simulink model "triplex_12B_with_contracts_PP"  (R2019b)
settings: Solver=FixedStepDiscrete  StartTime=0.0  StopTime=10.0  FixedStep=0.100000  RelTol=1e-3  EnableMultiTasking=on
model workspace (MAT data in the model file):
  ContractValidatorBlocksMap = containers.Map
  ContractValidatorBlocksMap.serialization.keys = {'triplex_12B/triplex_12B_TriplexSignalMonitorSpec/validator', 'triplex_12B_with_contracts/triplex_12B_TriplexSignalMonitorSpec/validator'}
  ContractValidatorBlocksMap.serialization.values{1}.block = 'triplex_12B/triplex_12B_TriplexSignalMonitorSpec/validator'
  ContractValidatorBlocksMap.serialization.values{1}.assumePorts = 1
  ContractValidatorBlocksMap.serialization.values{1}.guaranteePorts = 6
  ContractValidatorBlocksMap.serialization.values{1}.modeBlocksPorts = 0
  ContractValidatorBlocksMap.serialization.values{1}.portHandles.Inport = [1173.00195312 1174.00195312 1175.00195312 1176.00195312 1177.00195312 1178.00195312 1179.00195312]
  ContractValidatorBlocksMap.serialization.values{1}.portHandles.Outport = 1180.00195312
  ContractValidatorBlocksMap.serialization.values{1}.portHandles.Enable = []
  ContractValidatorBlocksMap.serialization.values{1}.portHandles.Trigger = []
  ContractValidatorBlocksMap.serialization.values{1}.portHandles.State = []
  ContractValidatorBlocksMap.serialization.values{1}.portHandles.LConn = []
  ContractValidatorBlocksMap.serialization.values{1}.portHandles.RConn = []
  ContractValidatorBlocksMap.serialization.values{1}.portHandles.Ifaction = []
  ContractValidatorBlocksMap.serialization.values{1}.portHandles.Reset = []
  ContractValidatorBlocksMap.serialization.values{1}.portConnectivity(1).Type = '1'
  ContractValidatorBlocksMap.serialization.values{1}.portConnectivity(1).Position = [365 -135]
  ContractValidatorBlocksMap.serialization.values{1}.portConnectivity(1).SrcBlock = 5288.00085449
  ContractValidatorBlocksMap.serialization.values{1}.portConnectivity(1).SrcPort = 0
  ContractValidatorBlocksMap.serialization.values{1}.portConnectivity(1).DstBlock = []
  ContractValidatorBlocksMap.serialization.values{1}.portConnectivity(1).DstPort = []
  ContractValidatorBlocksMap.serialization.values{1}.portConnectivity(2).Type = '2'
  ContractValidatorBlocksMap.serialization.values{1}.portConnectivity(2).Position = [365 -65]
  ContractValidatorBlocksMap.serialization.values{1}.portConnectivity(2).SrcBlock = 600.002807617
  ContractValidatorBlocksMap.serialization.values{1}.portConnectivity(2).SrcPort = 0
  ContractValidatorBlocksMap.serialization.values{1}.portConnectivity(2).DstBlock = []
  ContractValidatorBlocksMap.serialization.values{1}.portConnectivity(2).DstPort = []
  ContractValidatorBlocksMap.serialization.values{1}.portConnectivity(3).Type = '3'
  ContractValidatorBlocksMap.serialization.values{1}.portConnectivity(3).Position = [365 5]
  ContractValidatorBlocksMap.serialization.values{1}.portConnectivity(3).SrcBlock = 604.003051758
  ContractValidatorBlocksMap.serialization.values{1}.portConnectivity(3).SrcPort = 0
  ContractValidatorBlocksMap.serialization.values{1}.portConnectivity(3).DstBlock = []
  ContractValidatorBlocksMap.serialization.values{1}.portConnectivity(3).DstPort = []
  ContractValidatorBlocksMap.serialization.values{1}.portConnectivity(4).Type = '4'
  ContractValidatorBlocksMap.serialization.values{1}.portConnectivity(4).Position = [365 75]
  ContractValidatorBlocksMap.serialization.values{1}.portConnectivity(4).SrcBlock = 608.003051758
  ContractValidatorBlocksMap.serialization.values{1}.portConnectivity(4).SrcPort = 0
  ContractValidatorBlocksMap.serialization.values{1}.portConnectivity(4).DstBlock = []
  ContractValidatorBlocksMap.serialization.values{1}.portConnectivity(4).DstPort = []
  ContractValidatorBlocksMap.serialization.values{1}.portConnectivity(5).Type = '5'
  ContractValidatorBlocksMap.serialization.values{1}.portConnectivity(5).Position = [365 145]
  ContractValidatorBlocksMap.serialization.values{1}.portConnectivity(5).SrcBlock = 612.003051758
  ContractValidatorBlocksMap.serialization.values{1}.portConnectivity(5).SrcPort = 0
  ContractValidatorBlocksMap.serialization.values{1}.portConnectivity(5).DstBlock = []
  ContractValidatorBlocksMap.serialization.values{1}.portConnectivity(5).DstPort = []
  ContractValidatorBlocksMap.serialization.values{1}.portConnectivity(6).Type = '6'
  ContractValidatorBlocksMap.serialization.values{1}.portConnectivity(6).Position = [365 215]
  ContractValidatorBlocksMap.serialization.values{1}.portConnectivity(6).SrcBlock = 616.003051758
  ContractValidatorBlocksMap.serialization.values{1}.portConnectivity(6).SrcPort = 0
  ContractValidatorBlocksMap.serialization.values{1}.portConnectivity(6).DstBlock = []
  ContractValidatorBlocksMap.serialization.values{1}.portConnectivity(6).DstPort = []
  ContractValidatorBlocksMap.serialization.values{1}.portConnectivity(7).Type = '7'
  ContractValidatorBlocksMap.serialization.values{1}.portConnectivity(7).Position = [365 285]
  ContractValidatorBlocksMap.serialization.values{1}.portConnectivity(7).SrcBlock = 620.003051758
  ContractValidatorBlocksMap.serialization.values{1}.portConnectivity(7).SrcPort = 0
  ContractValidatorBlocksMap.serialization.values{1}.portConnectivity(7).DstBlock = []
  ContractValidatorBlocksMap.serialization.values{1}.portConnectivity(7).DstPort = []
  ContractValidatorBlocksMap.serialization.values{1}.portConnectivity(8).Type = '1'
  ContractValidatorBlocksMap.serialization.values{1}.portConnectivity(8).Position = [500 75]
  ContractValidatorBlocksMap.serialization.values{1}.portConnectivity(8).SrcBlock = []
  ContractValidatorBlocksMap.serialization.values{1}.portConnectivity(8).SrcPort = []
  ContractValidatorBlocksMap.serialization.values{1}.portConnectivity(8).DstBlock = 884.002807617
  ContractValidatorBlocksMap.serialization.values{1}.portConnectivity(8).DstPort = 0
  ContractValidatorBlocksMap.serialization.values{2}.block = 'triplex_12B_with_contracts/triplex_12B_TriplexSignalMonitorSpec/validator'
  ContractValidatorBlocksMap.serialization.values{2}.assumePorts = 0
  ContractValidatorBlocksMap.serialization.values{2}.guaranteePorts = 6
  ContractValidatorBlocksMap.serialization.values{2}.modeBlocksPorts = 0
  ContractValidatorBlocksMap.serialization.values{2}.portHandles.Inport = [2851.00195312 2852.0020752 2853.0020752 2854.00195312 2855.0020752 2856.00195312]
  ContractValidatorBlocksMap.serialization.values{2}.portHandles.Outport = 2857.0020752
  ContractValidatorBlocksMap.serialization.values{2}.portHandles.Enable = []
  ContractValidatorBlocksMap.serialization.values{2}.portHandles.Trigger = []
  ContractValidatorBlocksMap.serialization.values{2}.portHandles.State = []
  ContractValidatorBlocksMap.serialization.values{2}.portHandles.LConn = []
  ContractValidatorBlocksMap.serialization.values{2}.portHandles.RConn = []
  ContractValidatorBlocksMap.serialization.values{2}.portHandles.Ifaction = []
  ContractValidatorBlocksMap.serialization.values{2}.portHandles.Reset = []
  ContractValidatorBlocksMap.serialization.values{2}.portConnectivity(1).Type = '1'
  ContractValidatorBlocksMap.serialization.values{2}.portConnectivity(1).Position = [14780 -135]
  ContractValidatorBlocksMap.serialization.values{2}.portConnectivity(1).SrcBlock = 1443.00415039
  ContractValidatorBlocksMap.serialization.values{2}.portConnectivity(1).SrcPort = 0
  ContractValidatorBlocksMap.serialization.values{2}.portConnectivity(1).DstBlock = []
  ContractValidatorBlocksMap.serialization.values{2}.portConnectivity(1).DstPort = []
  ContractValidatorBlocksMap.serialization.values{2}.portConnectivity(2).Type = '2'
  ContractValidatorBlocksMap.serialization.values{2}.portConnectivity(2).Position = [14780 -50]
  ContractValidatorBlocksMap.serialization.values{2}.portConnectivity(2).SrcBlock = 1423.00378418
  ContractValidatorBlocksMap.serialization.values{2}.portConnectivity(2).SrcPort = 0
  ContractValidatorBlocksMap.serialization.values{2}.portConnectivity(2).DstBlock = []
  ContractValidatorBlocksMap.serialization.values{2}.portConnectivity(2).DstPort = []
  ContractValidatorBlocksMap.serialization.values{2}.portConnectivity(3).Type = '3'
  ContractValidatorBlocksMap.serialization.values{2}.portConnectivity(3).Position = [14780 35]
  ContractValidatorBlocksMap.serialization.values{2}.portConnectivity(3).SrcBlock = 1435.00390625
  ContractValidatorBlocksMap.serialization.values{2}.portConnectivity(3).SrcPort = 0
  ContractValidatorBlocksMap.serialization.values{2}.portConnectivity(3).DstBlock = []
  ContractValidatorBlocksMap.serialization.values{2}.portConnectivity(3).DstPort = []
  ContractValidatorBlocksMap.serialization.values{2}.portConnectivity(4).Type = '4'
  ContractValidatorBlocksMap.serialization.values{2}.portConnectivity(4).Position = [14780 120]
  ContractValidatorBlocksMap.serialization.values{2}.portConnectivity(4).SrcBlock = 1439.00305176
  ContractValidatorBlocksMap.serialization.values{2}.portConnectivity(4).SrcPort = 0
  ContractValidatorBlocksMap.serialization.values{2}.portConnectivity(4).DstBlock = []
  ContractValidatorBlocksMap.serialization.values{2}.portConnectivity(4).DstPort = []
  ContractValidatorBlocksMap.serialization.values{2}.portConnectivity(5).Type = '5'
  ContractValidatorBlocksMap.serialization.values{2}.portConnectivity(5).Position = [14780 205]
  ContractValidatorBlocksMap.serialization.values{2}.portConnectivity(5).SrcBlock = 1427.00415039
  ContractValidatorBlocksMap.serialization.values{2}.portConnectivity(5).SrcPort = 0
  ContractValidatorBlocksMap.serialization.values{2}.portConnectivity(5).DstBlock = []
  ContractValidatorBlocksMap.serialization.values{2}.portConnectivity(5).DstPort = []
  ContractValidatorBlocksMap.serialization.values{2}.portConnectivity(6).Type = '6'
  ContractValidatorBlocksMap.serialization.values{2}.portConnectivity(6).Position = [14780 290]
  ContractValidatorBlocksMap.serialization.values{2}.portConnectivity(6).SrcBlock = 1431.00537109
  ContractValidatorBlocksMap.serialization.values{2}.portConnectivity(6).SrcPort = 0
  ContractValidatorBlocksMap.serialization.values{2}.portConnectivity(6).DstBlock = []
  ContractValidatorBlocksMap.serialization.values{2}.portConnectivity(6).DstPort = []
  ContractValidatorBlocksMap.serialization.values{2}.portConnectivity(7).Type = '1'
  ContractValidatorBlocksMap.serialization.values{2}.portConnectivity(7).Position = [14915 80]
  ContractValidatorBlocksMap.serialization.values{2}.portConnectivity(7).SrcBlock = []
  ContractValidatorBlocksMap.serialization.values{2}.portConnectivity(7).SrcPort = []
  ContractValidatorBlocksMap.serialization.values{2}.portConnectivity(7).DstBlock = 2601.0020752
  ContractValidatorBlocksMap.serialization.values{2}.portConnectivity(7).DstPort = 0
  ContractValidatorBlocksMap.serialization.uniformity = 0
  ContractValidatorBlocksMap.serialization.keyType = 'char'
  ContractValidatorBlocksMap.serialization.valueType = 'any'
  already_pp = 1
  compositionalMap.analysisNames = {'triplex_12B_with_contracts_PP/TriplexMonitorNoFail'}
  compositionalMap.compositionalOptions = {{''}}
  compositionalMap.selectedOptions = 1
  maskControlsMap = containers.Map
  maskControlsMap.serialization.keys = {'triplex_12B_with_contracts_PP/triplex_12B_TriplexSignalMonitorSpec/TSM_minus_004'}
  maskControlsMap.serialization.values = {{'Display_counter_example_as_signals', 'Display_counter_example_as_tables', 'Display_counter_example_as_HTML_tables', 'Generate_an_outer_model_for_the_counter_example', 'Generate_an_inner_model_for_the_counter_example'}}
  maskControlsMap.serialization.uniformity = 0
  maskControlsMap.serialization.keyType = 'char'
  maskControlsMap.serialization.valueType = 'any'
  nodeNameToBlockNameMap : containers.Map (value not decoded)
  verificationResults : object (value not decoded)
undefined symbols (not defined in the file): contractAfterSimulation, contractBeforeSimulation, ContractBlock, ContractGuaranteeBlock, ContractValidatorBlock, saveValidatorParameters
(part 1 of 2)
settings Model: Creator=elliocm  LastModifiedBy=hbourbou
settings DataIOCC: LimitDataPoints=on  SaveFormat=StructureWithTime  SignalLoggingSaveFormat=ModelDataLogs  ReturnWorkspaceOutputs=off
settings OptimizationCC: ExpressionDepthLimit=2147483647  LifeSpan=inf
settings DebuggingCC: AlgebraicLoopMsg=error  ArtificialAlgebraicLoopMsg=error  UnderspecifiedInitializationDetection=Classic  MergeDetectMultiDrivingBlocksExec=none  SolverPrmCheckMsg=warning  MultiTaskDSMMsg=warning  MultiTaskCondExecSysMsg=none  SingleTaskRateTransMsg=error  StateNameClashWarn=warning  SFUnexpectedBacktrackingDiag=warning  SFNoUnconditionalDefaultTransitionDiag=warning  SFExecutionAtInitializationDiag=none  ArithmeticOperatorsInVariantConditions=warning
settings HardwareCC: ProdBitPerPointer=32  ProdBitPerSizeT=32  ProdBitPerPtrDiffT=32  ProdLargestAtomicFloat=None  ProdIntDivRoundTo=Undefined  ProdEndianess=Unspecified  ProdWordSize=32  ProdHWDeviceType=32-bit Generic
settings ModelReferenceCC: PropagateSignalLabelsOutOfModel=off
settings SFSimCC: SimUseLocalCustomCode=off  CustomCodeUndefinedFunction=UseInterfaceOnly
settings RTWCC: RTWUseLocalCustomCode=off
settings CodeAppCC: StateflowObjectComments=on
settings GRTTargetCC: TargetLangStandard=C89/C90 (ANSI)  GeneratePreprocessorConditionals=Disable all
settings ConfigComp: CovMetricSettings=dw  CovHtmlReporting=on  CovSaveCumulativeToWorkspaceVar=on  CovSaveSingleToWorkspaceVar=on  CovExternalEMLEnable=off

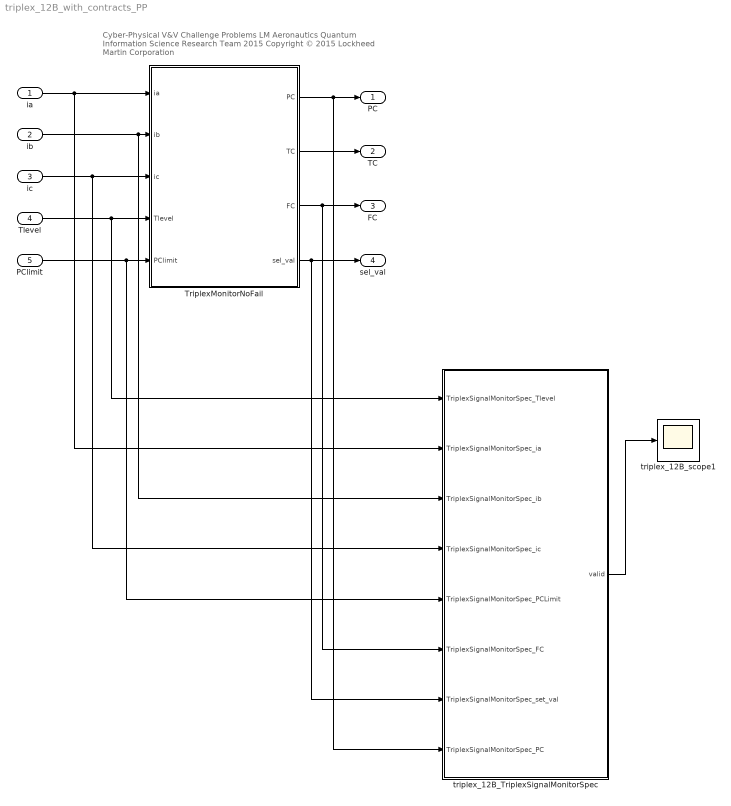
== system triplex_12B_with_contracts_PP ==
  note: Cyber-Physical V&V Challenge Problems
      | LM Aeronautics Quantum Information Science Research Team 2015
      | Copyright © 2015 Lockheed Martin Corporation
  ia : Inport  OutDataTypeStr=double
  ib : Inport  Port=2  OutDataTypeStr=double
  ic : Inport  Port=3  OutDataTypeStr=double
  Tlevel : Inport  Port=4  OutDataTypeStr=double
  PClimit : Inport  Port=5  OutDataTypeStr=int32
  TriplexMonitorNoFail : Subsystem  TreatAsAtomicUnit=on
  triplex_12B_TriplexSignalMonitorSpec : Subsystem  TreatAsAtomicUnit=on  mask(ContractBlock){ContractBlockType=ContractBlock}
      mask init:
      | set_param(gcb, 'LinkStatus', 'none');
      mask DialogControl DescTextVar Prompt: Contract block
      mask Display:
      | text(0.5, 0.5, '{\bf\fontsize{20}Contract}', 'hor', 'center', 'texmode','on');
      | blocks = find_system(gcb, 'LookUnderMasks','all', 'SearchDepth',1,'BlockType','Inport');
      | for i = 1 : length(blocks)
      |     blockName = get_param(blocks(i), 'Name');
      |     [path, blockName] = fileparts(char(blockName));
      |     port_label('input', i, blockName);
      | end
      | 
      | blocks = find_system(gcb, 'LookUnderMasks','all', 'SearchDepth',1,'BlockType','Outport');
      | for i = 1 : length(blocks)
      |     blockName = get_param(blocks(i), 'Name');
      |     [path, blockName] = fileparts(char(blockName));
      |     port_label('output', i, blockName);
      | end
  triplex_12B_scope1 : Scope
  PC : Outport  VectorParamsAs1DForOutWhenUnconnected=off
  TC : Outport  Port=2  VectorParamsAs1DForOutWhenUnconnected=off
  FC : Outport  Port=3  VectorParamsAs1DForOutWhenUnconnected=off
  sel_val : Outport  Port=4  VectorParamsAs1DForOutWhenUnconnected=off
  wires:
  ia/1 -> TriplexMonitorNoFail/1(ia), triplex_12B_TriplexSignalMonitorSpec/2(TriplexSignalMonitorSpec_ia)
  ib/1 -> TriplexMonitorNoFail/2(ib), triplex_12B_TriplexSignalMonitorSpec/3(TriplexSignalMonitorSpec_ib)
  Tlevel/1 -> TriplexMonitorNoFail/4(Tlevel), triplex_12B_TriplexSignalMonitorSpec/1(TriplexSignalMonitorSpec_Tlevel)
  PClimit/1 -> TriplexMonitorNoFail/5(PClimit), triplex_12B_TriplexSignalMonitorSpec/5(TriplexSignalMonitorSpec_PCLimit)
  TriplexMonitorNoFail/2(TC) -> TC/1
  TriplexMonitorNoFail/1(PC) -> PC/1, triplex_12B_TriplexSignalMonitorSpec/8(TriplexSignalMonitorSpec_PC)
  TriplexMonitorNoFail/4(sel_val) -> sel_val/1, triplex_12B_TriplexSignalMonitorSpec/7(TriplexSignalMonitorSpec_set_val)
  ic/1 -> TriplexMonitorNoFail/3(ic), triplex_12B_TriplexSignalMonitorSpec/4(TriplexSignalMonitorSpec_ic)
  TriplexMonitorNoFail/3(FC) -> FC/1, triplex_12B_TriplexSignalMonitorSpec/6(TriplexSignalMonitorSpec_FC)
  triplex_12B_TriplexSignalMonitorSpec/1(valid) -> triplex_12B_scope1/1

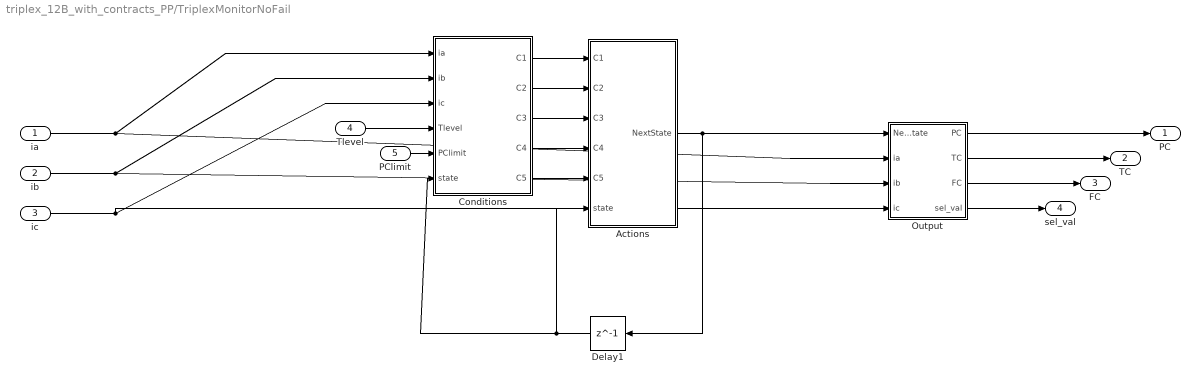
== system triplex_12B_with_contracts_PP/TriplexMonitorNoFail ==
  ia : Inport
  ib : Inport  Port=2
  ic : Inport  Port=3
  Tlevel : Inport  Port=4
  PClimit : Inport  Port=5
  Actions : Subsystem  TreatAsAtomicUnit=on
  Conditions : Subsystem  TreatAsAtomicUnit=on
  Delay1 : Delay  DelayLength=1  InitialCondition=0
  Output : Subsystem  TreatAsAtomicUnit=on
  PC : Outport  VectorParamsAs1DForOutWhenUnconnected=off
  TC : Outport  Port=2  VectorParamsAs1DForOutWhenUnconnected=off
  FC : Outport  Port=3  VectorParamsAs1DForOutWhenUnconnected=off
  sel_val : Outport  Port=4  VectorParamsAs1DForOutWhenUnconnected=off
  wires:
  Conditions/2(C2) -> Actions/2(C2)
  Conditions/5(C5) -> Actions/5(C5)
  Conditions/1(C1) -> Actions/1(C1)
  Conditions/4(C4) -> Actions/4(C4)
  Conditions/3(C3) -> Actions/3(C3)
  Tlevel/1 -> Conditions/4(Tlevel)
  PClimit/1 -> Conditions/5(PClimit)
  Output/2(TC) -> TC/1
  Output/1(PC) -> PC/1
  Output/3(FC) -> FC/1
  Actions/1(NextState) -> Delay1/1, Output/1(NextState)
  Delay1/1 -> Actions/6(state), Conditions/6(state)
  ia/1 -> Conditions/1(ia), Output/2(ia)
  ib/1 -> Conditions/2(ib), Output/3(ib)
  ic/1 -> Conditions/3(ic), Output/4(ic)
  Output/4(sel_val) -> sel_val/1

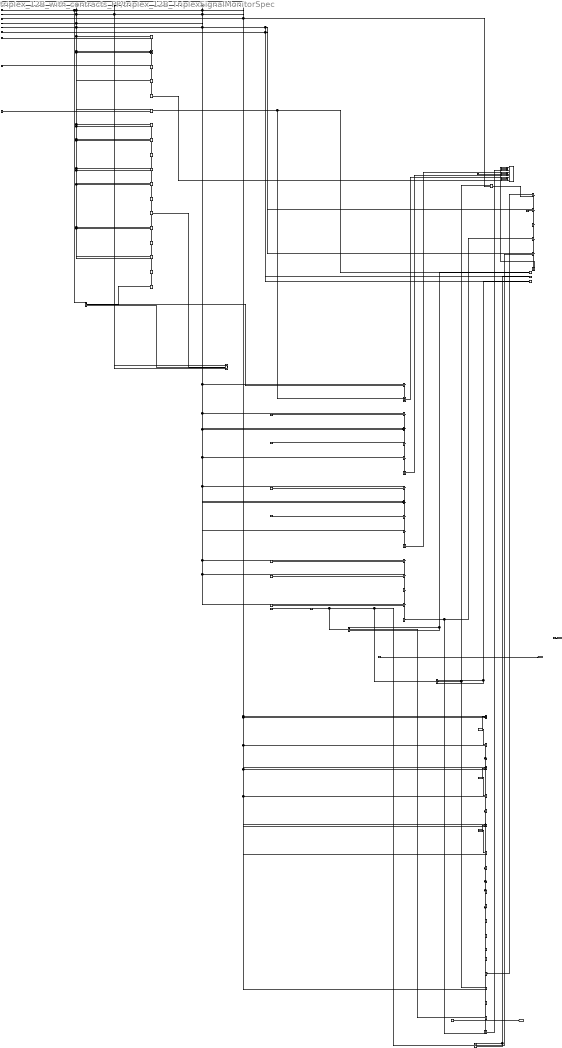
== system triplex_12B_with_contracts_PP/triplex_12B_TriplexSignalMonitorSpec ==
  TriplexSignalMonitorSpec_Tlevel : Inport  OutDataTypeStr=double
  TriplexSignalMonitorSpec_ia : Inport  Port=2  OutDataTypeStr=double
  TriplexSignalMonitorSpec_ib : Inport  Port=3  OutDataTypeStr=double
  TriplexSignalMonitorSpec_ic : Inport  Port=4  OutDataTypeStr=double
  TriplexSignalMonitorSpec_PCLimit : Inport  Port=5
  TriplexSignalMonitorSpec_FC : Inport  Port=6
  TriplexSignalMonitorSpec_set_val : Inport  Port=7  OutDataTypeStr=double
  TriplexSignalMonitorSpec_PC : Inport  Port=8
  Arrow_xxTriplexS_443436564_ec_35_ni_0 : Delay  DelayLength=1  InitialCondition=1
  C1_operator : RelationalOperator  Operator=>  OutDataTypeStr=boolean  RndMeth=Simplest
  C2_operator : RelationalOperator  Operator=>  OutDataTypeStr=boolean  RndMeth=Simplest
  C3_operator : RelationalOperator  Operator=>  OutDataTypeStr=boolean  RndMeth=Simplest
  PRE_xxTriplexSignalMonitorSpec_37 : Delay  DelayLength=1  InitialCondition=0
  PRE_xxTriplexSignalMonitorSpec_40 : Delay  DelayLength=1  InitialCondition=0
  PRE_xxTriplexSignalMonitorSpec_46 : Delay  DelayLength=1  InitialCondition=0
  TSM_minus_001 : Subsystem  TreatAsAtomicUnit=on  mask(ContractGuaranteeBlock){ContractBlockType=ContractGuaranteeBlock}
      mask init:
      | set_param(gcb, 'LinkStatus', 'none');
      mask DialogControl DescTextVar Prompt: Guarantee block
  TSM_minus_002 : Subsystem  TreatAsAtomicUnit=on  mask(ContractGuaranteeBlock){ContractBlockType=ContractGuaranteeBlock}
      mask init:
      | set_param(gcb, 'LinkStatus', 'none');
      mask DialogControl DescTextVar Prompt: Guarantee block
  TSM_minus_003a : Subsystem  TreatAsAtomicUnit=on  mask(ContractGuaranteeBlock){ContractBlockType=ContractGuaranteeBlock}
      mask init:
      | set_param(gcb, 'LinkStatus', 'none');
      mask DialogControl DescTextVar Prompt: Guarantee block
  TSM_minus_003b : Subsystem  TreatAsAtomicUnit=on  mask(ContractGuaranteeBlock){ContractBlockType=ContractGuaranteeBlock}
      mask init:
      | set_param(gcb, 'LinkStatus', 'none');
      mask DialogControl DescTextVar Prompt: Guarantee block
  TSM_minus_003c : Subsystem  TreatAsAtomicUnit=on  mask(ContractGuaranteeBlock){ContractBlockType=ContractGuaranteeBlock}
      mask init:
      | set_param(gcb, 'LinkStatus', 'none');
      mask DialogControl DescTextVar Prompt: Guarantee block
  TSM_minus_004 : Subsystem  TreatAsAtomicUnit=on  mask(ContractGuaranteeBlock){ContractBlockType=ContractGuaranteeBlock}
      mask init:
      | set_param(gcb, 'LinkStatus', 'none');
      mask DialogControl DescTextVar Prompt: Guarantee block
      mask DialogControl Display_counter_example_as_signals Prompt: Display counter example as signals
      mask DialogControl Display_counter_example_as_signals Callback: displayCexSignals(1, 1);
      mask DialogControl Display_counter_example_as_tables Prompt: Display counter example as tables
      mask DialogControl Display_counter_example_as_tables Callback: displayCexTables(1, 1);
      mask DialogControl Display_counter_example_as_HTML_tables Prompt: Display counter example as HTML tables
      mask DialogControl Display_counter_example_as_HTML_tables Callback: displayCexHtmlTables(1, 1);
      mask DialogControl Generate_an_outer_model_for_the_counter_example Prompt: Generate an outer model for the counter example
      mask DialogControl Generate_an_outer_model_for_the_counter_example Callback: generateModelWithSignalBuilders(1, 1, 2);
      mask DialogControl Generate_an_inner_model_for_the_counter_example Prompt: Generate an inner model for the counter example
      mask DialogControl Generate_an_inner_model_for_the_counter_example Callback: generateModelWithSignalBuilders(1, 1, 1);
  abs_call : Subsystem  TreatAsAtomicUnit=on
  abs_call1 : Subsystem  TreatAsAtomicUnit=on
  abs_call11 : Subsystem  TreatAsAtomicUnit=on
  branch_10_IF : Switch  Criteria=u2 ~= 0
  branch_11_IF : Switch  Criteria=u2 ~= 0
  branch_12_IF : Switch  Criteria=u2 ~= 0
  branch_13_IF : Switch  Criteria=u2 ~= 0
  branch_9_IF : Switch  Criteria=u2 ~= 0
  failure_in_progress_operator : Logic  AllPortsSameDT=off  OutDataTypeStr=boolean
  failure_must_be_latched_operator : Logic  AllPortsSameDT=off  OutDataTypeStr=boolean
  miscompare_operator : Logic  Operator=OR  AllPortsSameDT=off  OutDataTypeStr=boolean
  no_fail_operator : RelationalOperator  Operator===  OutDataTypeStr=boolean  RndMeth=Simplest
  no_fail_rhs_2 : Constant  Value=0  OutDataTypeStr=int32
  single_fail_reported_operator : Logic  Operator=OR  AllPortsSameDT=off  OutDataTypeStr=boolean
  spec284_operator : Subsystem  TreatAsAtomicUnit=on
  spec292_operator : Subsystem  TreatAsAtomicUnit=on
  spec309_operator : Subsystem  TreatAsAtomicUnit=on
  spec326_operator : Subsystem  TreatAsAtomicUnit=on
  spec334_operator : Subsystem  TreatAsAtomicUnit=on
  spec351_operator : Subsystem  TreatAsAtomicUnit=on
  validator : M-S-Function  LoadFcn=saveValidatorParameters(gcb);  InitFcn=contractBeforeSimulation();  StopFcn=contractAfterSimulation();  FunctionName=contract  mask(ContractValidatorBlock){assumePorts=0, guaranteePorts=6, modePorts=0, ContractBlockType=ContractValidatorBlock, createInportsCheckbox=off}
      mask prompts: assumePorts "Assume ports     :"; guaranteePorts "Guarantee ports :"; modePorts "Mode ports        :"; createInportsCheckbox "Create inports and connect them automatically"
      mask init:
      | set_param(gcb,'LinkStatus','none');
      | contract_callback('inputs_callback',gcb);
      mask DialogControl DescTextVar Prompt: The validator block implements the following logic: <br> <br> <b>Sofar</b>(assume<sub>1</sub> <b>&#8743;</b> assume<sub>2</sub> <b>&#8743;</b> ... assume<sub>k</sub>) <b>&rarr;</b> (guarantee<sub>1</sub> <b>&#8743;</b> guarantee<sub>2</sub> <b>&#8743;</b> ... guarantee<sub>m</sub> <b>&#8743;</b>  mode<sub>1</sub> <b>&#8743;</b> mode<sub>2</sub> <b>&#8743;</b> ... <b>&#8743;</b> mode<sub>n</sub> )<br> where mode<sub>i</sub> = require<sub>i</sub> <b>&rarr;</b> ensure<sub>i</sub>
      mask Display:
      | color('black');
      | port_label('input',1,'guarantee');
      | port_label('input',2,'guarantee');
      | port_label('input',3,'guarantee');
      | port_label('input',4,'guarantee');
      | port_label('input',5,'guarantee');
      | port_label('input',6,'guarantee');
      | port_label('output',1,'valid');
  xxTriplexS_443436564_ec_35_ni_0_init : Constant  Value=0  OutDataTypeStr=boolean
  xxTriplexSignalMonitorSpec_10_operator : Sum  OutDataTypeStr=double
  xxTriplexSignalMonitorSpec_11_operator : Product  OutDataTypeStr=double
  xxTriplexSignalMonitorSpec_11_rhs_1 : Constant  Value=0.5  OutDataTypeStr=double
  xxTriplexSignalMonitorSpec_12_operator : RelationalOperator  Operator===  OutDataTypeStr=boolean  RndMeth=Simplest
  xxTriplexSignalMonitorSpec_13_operator : RelationalOperator  Operator===  OutDataTypeStr=boolean  RndMeth=Simplest
  xxTriplexSignalMonitorSpec_13_rhs_2 : Constant  Value=2  OutDataTypeStr=int32
  xxTriplexSignalMonitorSpec_14_operator : Logic  AllPortsSameDT=off  OutDataTypeStr=boolean
  xxTriplexSignalMonitorSpec_15_operator : RelationalOperator  Operator===  OutDataTypeStr=boolean  RndMeth=Simplest
  xxTriplexSignalMonitorSpec_16_operator : Logic  AllPortsSameDT=off  OutDataTypeStr=boolean
  xxTriplexSignalMonitorSpec_17_operator : Sum  Inputs=+-  OutDataTypeStr=double
  xxTriplexSignalMonitorSpec_19_operator : Sum  Inputs=+-  OutDataTypeStr=double
  xxTriplexSignalMonitorSpec_1_operator : Sum  OutDataTypeStr=double
  xxTriplexSignalMonitorSpec_21_operator : Sum  Inputs=+-  OutDataTypeStr=double
  xxTriplexSignalMonitorSpec_23_operator : RelationalOperator  Operator=<=  OutDataTypeStr=boolean  RndMeth=Simplest
  xxTriplexSignalMonitorSpec_24_operator : RelationalOperator  Operator=<=  OutDataTypeStr=boolean  RndMeth=Simplest
  xxTriplexSignalMonitorSpec_25_operator : Logic  AllPortsSameDT=off  OutDataTypeStr=boolean
  xxTriplexSignalMonitorSpec_26_operator : RelationalOperator  Operator=<=  OutDataTypeStr=boolean  RndMeth=Simplest
  xxTriplexSignalMonitorSpec_27_operator : RelationalOperator  Operator=<=  OutDataTypeStr=boolean  RndMeth=Simplest
  xxTriplexSignalMonitorSpec_28_operator : Logic  AllPortsSameDT=off  OutDataTypeStr=boolean
  xxTriplexSignalMonitorSpec_29_operator : Logic  Operator=OR  AllPortsSameDT=off  OutDataTypeStr=boolean
  xxTriplexSignalMonitorSpec_2_operator : Product  OutDataTypeStr=double
  xxTriplexSignalMonitorSpec_2_rhs_1 : Constant  Value=0.5  OutDataTypeStr=double
  xxTriplexSignalMonitorSpec_30_operator : RelationalOperator  Operator=<=  OutDataTypeStr=boolean  RndMeth=Simplest
  xxTriplexSignalMonitorSpec_31_operator : Logic  AllPortsSameDT=off  OutDataTypeStr=boolean
  xxTriplexSignalMonitorSpec_32_operator : RelationalOperator  Operator=<=  OutDataTypeStr=boolean  RndMeth=Simplest
  xxTriplexSignalMonitorSpec_33_operator : Logic  AllPortsSameDT=off  OutDataTypeStr=boolean
  xxTriplexSignalMonitorSpec_34_operator : Logic  Operator=OR  AllPortsSameDT=off  OutDataTypeStr=boolean
  xxTriplexSignalMonitorSpec_36_rhs : Constant  Value=0  OutDataTypeStr=Inherit: Inherit via back propagation
  xxTriplexSignalMonitorSpec_39_rhs : Constant  Value=0.0  OutDataTypeStr=double
  xxTriplexSignalMonitorSpec_3_operator : RelationalOperator  Operator===  OutDataTypeStr=boolean  RndMeth=Simplest
  xxTriplexSignalMonitorSpec_42_operator : RelationalOperator  Operator=>  OutDataTypeStr=boolean  RndMeth=Simplest
  xxTriplexSignalMonitorSpec_42_rhs_2 : Constant  Value=0  OutDataTypeStr=int32
  xxTriplexSignalMonitorSpec_43_operator : RelationalOperator  Operator=<=  OutDataTypeStr=boolean  RndMeth=Simplest
  xxTriplexSignalMonitorSpec_44_operator : Logic  AllPortsSameDT=off  OutDataTypeStr=boolean
  xxTriplexSignalMonitorSpec_45_operator : RelationalOperator  Operator=>  OutDataTypeStr=boolean  RndMeth=Simplest
  xxTriplexSignalMonitorSpec_47_rhs1 : Constant  Value=true  OutDataTypeStr=boolean
  xxTriplexSignalMonitorSpec_48_operator : RelationalOperator  Operator===  OutDataTypeStr=boolean  RndMeth=Simplest
  xxTriplexSignalMonitorSpec_48_rhs_2 : Constant  Value=4  OutDataTypeStr=int32
  xxTriplexSignalMonitorSpec_49_operator : RelationalOperator  Operator===  OutDataTypeStr=boolean  RndMeth=Simplest
  xxTriplexSignalMonitorSpec_49_rhs_2 : Constant  Value=2  OutDataTypeStr=int32
  xxTriplexSignalMonitorSpec_4_operator : RelationalOperator  Operator===  OutDataTypeStr=boolean  RndMeth=Simplest
  xxTriplexSignalMonitorSpec_4_rhs_2 : Constant  OutDataTypeStr=int32
  xxTriplexSignalMonitorSpec_50_operator : RelationalOperator  Operator===  OutDataTypeStr=boolean  RndMeth=Simplest
  xxTriplexSignalMonitorSpec_50_rhs_2 : Constant  OutDataTypeStr=int32
  xxTriplexSignalMonitorSpec_51_operator : Logic  Operator=OR  AllPortsSameDT=off  OutDataTypeStr=boolean
  xxTriplexSignalMonitorSpec_52_operator : Logic  Operator=NOT  AllPortsSameDT=off  OutDataTypeStr=boolean
  xxTriplexSignalMonitorSpec_53_operator : Logic  AllPortsSameDT=off  OutDataTypeStr=boolean
  xxTriplexSignalMonitorSpec_54_operator : Logic  AllPortsSameDT=off  OutDataTypeStr=boolean
  xxTriplexSignalMonitorSpec_55_operator : Logic  Operator=NOT  AllPortsSameDT=off  OutDataTypeStr=boolean
  xxTriplexSignalMonitorSpec_56_operator : Logic  AllPortsSameDT=off  OutDataTypeStr=boolean
  xxTriplexSignalMonitorSpec_57_operator : Logic  AllPortsSameDT=off  OutDataTypeStr=boolean
  xxTriplexSignalMonitorSpec_58_operator : Logic  Operator=NOT  AllPortsSameDT=off  OutDataTypeStr=boolean
  xxTriplexSignalMonitorSpec_59_operator : Logic  AllPortsSameDT=off  OutDataTypeStr=boolean
  xxTriplexSignalMonitorSpec_5_operator : RelationalOperator  Operator===  OutDataTypeStr=boolean  RndMeth=Simplest
  xxTriplexSignalMonitorSpec_60_operator : Logic  AllPortsSameDT=off  OutDataTypeStr=boolean
  xxTriplexSignalMonitorSpec_61_operator : Logic  Operator=OR  AllPortsSameDT=off  OutDataTypeStr=boolean
  xxTriplexSignalMonitorSpec_6_operator : Sum  OutDataTypeStr=double
  xxTriplexSignalMonitorSpec_7_operator : Product  OutDataTypeStr=double
  xxTriplexSignalMonitorSpec_7_rhs_1 : Constant  Value=0.5  OutDataTypeStr=double
  xxTriplexSignalMonitorSpec_8_operator : RelationalOperator  Operator===  OutDataTypeStr=boolean  RndMeth=Simplest
  xxTriplexSignalMonitorSpec_9_operator : RelationalOperator  Operator===  OutDataTypeStr=boolean  RndMeth=Simplest
  xxTriplexSignalMonitorSpec_9_rhs_2 : Constant  Value=4  OutDataTypeStr=int32
  valid : Outport
  wires:
  validator/1 -> valid/1
  xxTriplexSignalMonitorSpec_9_rhs_2/1 -> xxTriplexSignalMonitorSpec_9_operator/2
  xxTriplexSignalMonitorSpec_7_operator/1 -> xxTriplexSignalMonitorSpec_8_operator/2
  xxTriplexSignalMonitorSpec_6_operator/1 -> xxTriplexSignalMonitorSpec_7_operator/2
  xxTriplexSignalMonitorSpec_7_rhs_1/1 -> xxTriplexSignalMonitorSpec_7_operator/1
  xxTriplexSignalMonitorSpec_57_operator/1 -> xxTriplexSignalMonitorSpec_61_operator/2
  xxTriplexSignalMonitorSpec_60_operator/1 -> xxTriplexSignalMonitorSpec_61_operator/1
  xxTriplexSignalMonitorSpec_59_operator/1 -> xxTriplexSignalMonitorSpec_60_operator/1
  branch_9_IF/1 -> xxTriplexSignalMonitorSpec_5_operator/2
  xxTriplexSignalMonitorSpec_58_operator/1 -> xxTriplexSignalMonitorSpec_59_operator/1
  xxTriplexSignalMonitorSpec_56_operator/1 -> xxTriplexSignalMonitorSpec_57_operator/1
  xxTriplexSignalMonitorSpec_55_operator/1 -> xxTriplexSignalMonitorSpec_56_operator/2
  xxTriplexSignalMonitorSpec_52_operator/1 -> xxTriplexSignalMonitorSpec_54_operator/2
  xxTriplexSignalMonitorSpec_53_operator/1 -> xxTriplexSignalMonitorSpec_54_operator/1
  xxTriplexSignalMonitorSpec_49_operator/1 -> xxTriplexSignalMonitorSpec_51_operator/2
  xxTriplexSignalMonitorSpec_50_operator/1 -> xxTriplexSignalMonitorSpec_51_operator/1
  xxTriplexSignalMonitorSpec_50_rhs_2/1 -> xxTriplexSignalMonitorSpec_50_operator/2
  xxTriplexSignalMonitorSpec_4_rhs_2/1 -> xxTriplexSignalMonitorSpec_4_operator/2
  xxTriplexSignalMonitorSpec_49_rhs_2/1 -> xxTriplexSignalMonitorSpec_49_operator/2
  xxTriplexSignalMonitorSpec_48_rhs_2/1 -> xxTriplexSignalMonitorSpec_48_operator/2
  xxTriplexSignalMonitorSpec_47_rhs1/1 -> [a_e_xxTriplexSignalMonitorSpec_47]
  xxTriplexSignalMonitorSpec_43_operator/1 -> xxTriplexSignalMonitorSpec_44_operator/2
  xxTriplexSignalMonitorSpec_42_rhs_2/1 -> xxTriplexSignalMonitorSpec_42_operator/2
  xxTriplexSignalMonitorSpec_39_rhs/1 -> [a_e_xxTriplexSignalMonitorSpec_41]
  xxTriplexSignalMonitorSpec_2_operator/1 -> xxTriplexSignalMonitorSpec_3_operator/2
  xxTriplexSignalMonitorSpec_36_rhs/1 -> [a_e_xxTriplexSignalMonitorSpec_38]
  xxTriplexSignalMonitorSpec_31_operator/1 -> xxTriplexSignalMonitorSpec_34_operator/2
  xxTriplexSignalMonitorSpec_33_operator/1 -> xxTriplexSignalMonitorSpec_34_operator/1
  xxTriplexSignalMonitorSpec_32_operator/1 -> xxTriplexSignalMonitorSpec_33_operator/2
  xxTriplexSignalMonitorSpec_30_operator/1 -> xxTriplexSignalMonitorSpec_31_operator/1
  xxTriplexSignalMonitorSpec_1_operator/1 -> xxTriplexSignalMonitorSpec_2_operator/2
  xxTriplexSignalMonitorSpec_2_rhs_1/1 -> xxTriplexSignalMonitorSpec_2_operator/1
  xxTriplexSignalMonitorSpec_25_operator/1 -> xxTriplexSignalMonitorSpec_29_operator/2
  xxTriplexSignalMonitorSpec_28_operator/1 -> xxTriplexSignalMonitorSpec_29_operator/1
  xxTriplexSignalMonitorSpec_26_operator/1 -> xxTriplexSignalMonitorSpec_28_operator/2
  xxTriplexSignalMonitorSpec_24_operator/1 -> xxTriplexSignalMonitorSpec_25_operator/1
  failure_in_progress_operator/1 -> xxTriplexSignalMonitorSpec_16_operator/2
  branch_13_IF/1 -> xxTriplexSignalMonitorSpec_15_operator/2
  failure_must_be_latched_operator/1 -> xxTriplexSignalMonitorSpec_14_operator/2
  branch_11_IF/1 -> xxTriplexSignalMonitorSpec_14_operator/1
  xxTriplexSignalMonitorSpec_13_rhs_2/1 -> xxTriplexSignalMonitorSpec_13_operator/2
  xxTriplexSignalMonitorSpec_11_operator/1 -> xxTriplexSignalMonitorSpec_12_operator/2
  xxTriplexSignalMonitorSpec_10_operator/1 -> xxTriplexSignalMonitorSpec_11_operator/2
  xxTriplexSignalMonitorSpec_11_rhs_1/1 -> xxTriplexSignalMonitorSpec_11_operator/1
  TSM_minus_003a/1(guarantee) -> validator/6
  TSM_minus_002/1(guarantee) -> validator/5
  TSM_minus_003c/1(guarantee) -> validator/4
  TSM_minus_003b/1(guarantee) -> validator/3
  TSM_minus_001/1(guarantee) -> validator/2
  TSM_minus_004/1(guarantee) -> validator/1
  xxTriplexSignalMonitorSpec_3_operator/1 -> spec351_operator/2(B)
  xxTriplexSignalMonitorSpec_4_operator/1 -> spec351_operator/1(A)
  xxTriplexSignalMonitorSpec_5_operator/1 -> spec334_operator/2(B)
  xxTriplexSignalMonitorSpec_8_operator/1 -> spec326_operator/2(B)
  xxTriplexSignalMonitorSpec_9_operator/1 -> spec326_operator/1(A)
  xxTriplexSignalMonitorSpec_12_operator/1 -> spec309_operator/2(B)
  xxTriplexSignalMonitorSpec_13_operator/1 -> spec309_operator/1(A)
  xxTriplexSignalMonitorSpec_14_operator/1 -> spec292_operator/1(A)
  xxTriplexSignalMonitorSpec_15_operator/1 -> spec284_operator/2(B)
  xxTriplexSignalMonitorSpec_16_operator/1 -> spec284_operator/1(A)
  xxTriplexSignalMonitorSpec_48_operator/1 -> single_fail_reported_operator/2
  xxTriplexSignalMonitorSpec_51_operator/1 -> single_fail_reported_operator/1
  no_fail_rhs_2/1 -> no_fail_operator/2
  xxTriplexSignalMonitorSpec_54_operator/1 -> miscompare_operator/2
  xxTriplexSignalMonitorSpec_61_operator/1 -> miscompare_operator/1
  spec351_operator/1(A_equal__equal__gt_B) -> TSM_minus_003a/1(In1)
  spec334_operator/1(A_equal__equal__gt_B) -> TSM_minus_002/1(In1)
  spec326_operator/1(A_equal__equal__gt_B) -> TSM_minus_003c/1(In1)
  spec309_operator/1(A_equal__equal__gt_B) -> TSM_minus_003b/1(In1)
  spec292_operator/1(A_equal__equal__gt_B) -> TSM_minus_001/1(In1)
  spec284_operator/1(A_equal__equal__gt_B) -> TSM_minus_004/1(In1)
  xxTriplexSignalMonitorSpec_45_operator/1 -> failure_must_be_latched_operator/2
  xxTriplexSignalMonitorSpec_42_operator/1 -> failure_in_progress_operator/2
  xxTriplexSignalMonitorSpec_44_operator/1 -> failure_in_progress_operator/1
  branch_10_IF/1 -> branch_9_IF/3
  xxTriplexSignalMonitorSpec_29_operator/1 -> branch_9_IF/2
  xxTriplexSignalMonitorSpec_34_operator/1 -> branch_10_IF/2
  xxTriplexSignalMonitorSpec_21_operator/1 -> abs_call11/1(abs_x)
  xxTriplexSignalMonitorSpec_19_operator/1 -> abs_call1/1(abs_x)
  xxTriplexSignalMonitorSpec_17_operator/1 -> abs_call/1(abs_x)
  abs_call11/1(abs_y) -> C3_operator/1
  abs_call1/1(abs_y) -> C2_operator/1
  abs_call/1(abs_y) -> C1_operator/1
  xxTriplexS_443436564_ec_35_ni_0_init/1 -> Arrow_xxTriplexS_443436564_ec_35_ni_0/1
  TriplexSignalMonitorSpec_PC/1 -> xxTriplexSignalMonitorSpec_42_operator/1, PRE_xxTriplexSignalMonitorSpec_37/1
  TriplexSignalMonitorSpec_PCLimit/1 -> xxTriplexSignalMonitorSpec_45_operator/2, xxTriplexSignalMonitorSpec_43_operator/2
  branch_12_IF/1 -> xxTriplexSignalMonitorSpec_45_operator/1, xxTriplexSignalMonitorSpec_43_operator/1
  PRE_xxTriplexSignalMonitorSpec_40/1 -> branch_13_IF/3, branch_13_IF/1
  single_fail_reported_operator/1 -> xxTriplexSignalMonitorSpec_16_operator/1, spec292_operator/2(B)
  miscompare_operator/1 -> xxTriplexSignalMonitorSpec_44_operator/1, failure_must_be_latched_operator/1
  C3_operator/1 -> xxTriplexSignalMonitorSpec_57_operator/2, xxTriplexSignalMonitorSpec_52_operator/1, xxTriplexSignalMonitorSpec_60_operator/2
  C2_operator/1 -> xxTriplexSignalMonitorSpec_55_operator/1, xxTriplexSignalMonitorSpec_53_operator/2, xxTriplexSignalMonitorSpec_59_operator/2
  C1_operator/1 -> xxTriplexSignalMonitorSpec_56_operator/1, xxTriplexSignalMonitorSpec_53_operator/1, xxTriplexSignalMonitorSpec_58_operator/1
  TriplexSignalMonitorSpec_Tlevel/1 -> C3_operator/2, C2_operator/2, C1_operator/2
  PRE_xxTriplexSignalMonitorSpec_37/1 -> branch_12_IF/3, branch_12_IF/1
  Arrow_xxTriplexS_443436564_ec_35_ni_0/1 -> branch_13_IF/2, branch_12_IF/2, branch_11_IF/2
  PRE_xxTriplexSignalMonitorSpec_46/1 -> branch_11_IF/3, branch_11_IF/1
  TriplexSignalMonitorSpec_set_val/1 -> xxTriplexSignalMonitorSpec_8_operator/1, xxTriplexSignalMonitorSpec_12_operator/1, xxTriplexSignalMonitorSpec_5_operator/1, xxTriplexSignalMonitorSpec_15_operator/1, PRE_xxTriplexSignalMonitorSpec_40/1, xxTriplexSignalMonitorSpec_3_operator/1
  no_fail_operator/1 -> spec334_operator/1(A), PRE_xxTriplexSignalMonitorSpec_46/1
  TriplexSignalMonitorSpec_ia/1 -> xxTriplexSignalMonitorSpec_30_operator/2, xxTriplexSignalMonitorSpec_27_operator/1, xxTriplexSignalMonitorSpec_23_operator/2, xxTriplexSignalMonitorSpec_32_operator/1, xxTriplexSignalMonitorSpec_1_operator/1, xxTriplexSignalMonitorSpec_21_operator/1, xxTriplexSignalMonitorSpec_17_operator/1, xxTriplexSignalMonitorSpec_10_operator/1, branch_10_IF/1
  TriplexSignalMonitorSpec_ib/1 -> xxTriplexSignalMonitorSpec_26_operator/1, xxTriplexSignalMonitorSpec_24_operator/2, xxTriplexSignalMonitorSpec_27_operator/2, xxTriplexSignalMonitorSpec_23_operator/1, xxTriplexSignalMonitorSpec_1_operator/2, xxTriplexSignalMonitorSpec_19_operator/1, xxTriplexSignalMonitorSpec_17_operator/2, xxTriplexSignalMonitorSpec_6_operator/1, branch_9_IF/1
  TriplexSignalMonitorSpec_ic/1 -> xxTriplexSignalMonitorSpec_26_operator/2, xxTriplexSignalMonitorSpec_24_operator/1, xxTriplexSignalMonitorSpec_30_operator/1, xxTriplexSignalMonitorSpec_32_operator/2, xxTriplexSignalMonitorSpec_6_operator/2, xxTriplexSignalMonitorSpec_10_operator/2, xxTriplexSignalMonitorSpec_21_operator/2, xxTriplexSignalMonitorSpec_19_operator/2, branch_10_IF/3
  xxTriplexSignalMonitorSpec_23_operator/1 -> xxTriplexSignalMonitorSpec_33_operator/1, xxTriplexSignalMonitorSpec_25_operator/2
  xxTriplexSignalMonitorSpec_27_operator/1 -> xxTriplexSignalMonitorSpec_31_operator/2, xxTriplexSignalMonitorSpec_28_operator/1
  TriplexSignalMonitorSpec_FC/1 -> xxTriplexSignalMonitorSpec_4_operator/1, no_fail_operator/1, xxTriplexSignalMonitorSpec_49_operator/1, xxTriplexSignalMonitorSpec_48_operator/1, xxTriplexSignalMonitorSpec_50_operator/1, xxTriplexSignalMonitorSpec_13_operator/1, xxTriplexSignalMonitorSpec_9_operator/1

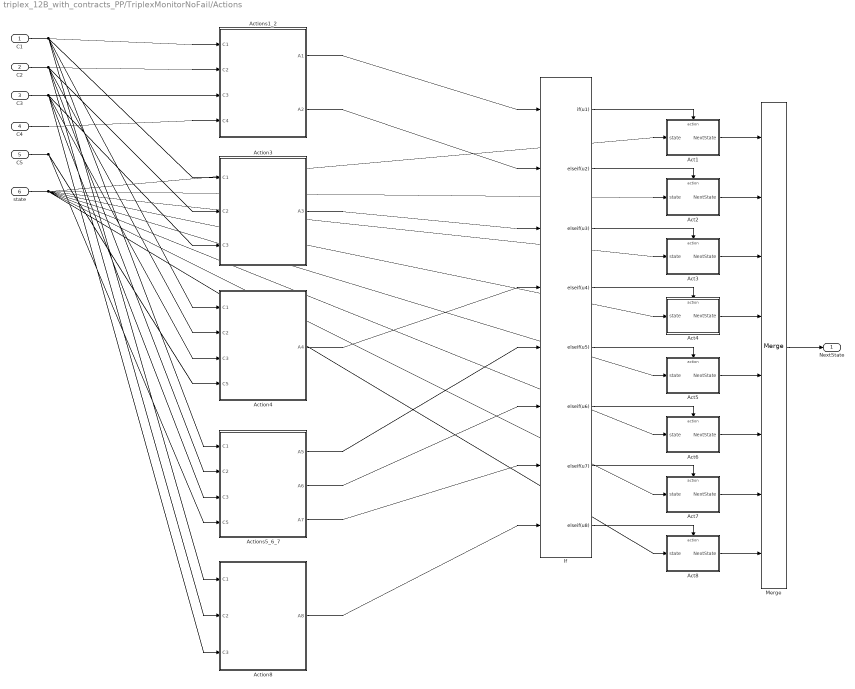
== system triplex_12B_with_contracts_PP/TriplexMonitorNoFail/Actions ==
  C1 : Inport
  C2 : Inport  Port=2
  C3 : Inport  Port=3
  C4 : Inport  Port=4
  C5 : Inport  Port=5
  state : Inport  Port=6
  Act1 : Subsystem  TreatAsAtomicUnit=on
  Act2 : Subsystem  TreatAsAtomicUnit=on
  Act3 : Subsystem  TreatAsAtomicUnit=on
  Act4 : Subsystem  TreatAsAtomicUnit=on
  Act5 : Subsystem  TreatAsAtomicUnit=on
  Act6 : Subsystem  TreatAsAtomicUnit=on
  Act7 : Subsystem  TreatAsAtomicUnit=on
  Act8 : Subsystem  TreatAsAtomicUnit=on
  Action3 : Subsystem  TreatAsAtomicUnit=on
  Action4 : Subsystem  TreatAsAtomicUnit=on
  Action8 : Subsystem  TreatAsAtomicUnit=on
  Actions1_2 : Subsystem  TreatAsAtomicUnit=on
  Actions5_6_7 : Subsystem  TreatAsAtomicUnit=on
  If : If  NumInputs=8  IfExpression=u1  ElseIfExpressions=u2, u3, u4, u5, u6, u7, u8  ShowElse=off
  Merge : Merge  Inputs=8
  NextState : Outport  VectorParamsAs1DForOutWhenUnconnected=off
  wires:
  C4/1 -> Actions1_2/4(C4)
  C3/1 -> Actions1_2/3(C3), Actions5_6_7/3(C3), Action8/3(C3), Action3/3(C3), Action4/3(C3)
  C2/1 -> Action4/2(C2), Actions5_6_7/2(C2), Action8/2(C2), Actions1_2/2(C2), Action3/2(C2)
  C5/1 -> Action4/4(C5), Actions5_6_7/4(C5)
  C1/1 -> Actions5_6_7/1(C1), Action8/1(C1), Actions1_2/1(C1), Action3/1(C1), Action4/1(C1)
  Actions1_2/1(A1) -> If/1
  If/1 -> Act1/Action
  Actions1_2/2(A2) -> If/2
  If/2 -> Act2/Action
  If/3 -> Act3/Action
  Action3/1(A3) -> If/3
  Action4/1(A4) -> If/4
  Actions5_6_7/1(A5) -> If/5
  Actions5_6_7/2(A6) -> If/6
  Actions5_6_7/3(A7) -> If/7
  Action8/1(A8) -> If/8
  If/4 -> Act4/Action
  If/5 -> Act5/Action
  If/6 -> Act6/Action
  If/7 -> Act7/Action
  If/8 -> Act8/Action
  Act1/1(NextState) -> Merge/1
  Act2/1(NextState) -> Merge/2
  Act3/1(NextState) -> Merge/3
  Act4/1(NextState) -> Merge/4
  Act5/1(NextState) -> Merge/5
  Act6/1(NextState) -> Merge/6
  Act7/1(NextState) -> Merge/7
  Act8/1(NextState) -> Merge/8
  Merge/1 -> NextState/1
  state/1 -> Act2/1(state), Act3/1(state), Act4/1(state), Act1/1(state), Act5/1(state), Act6/1(state), Act7/1(state), Act8/1(state)

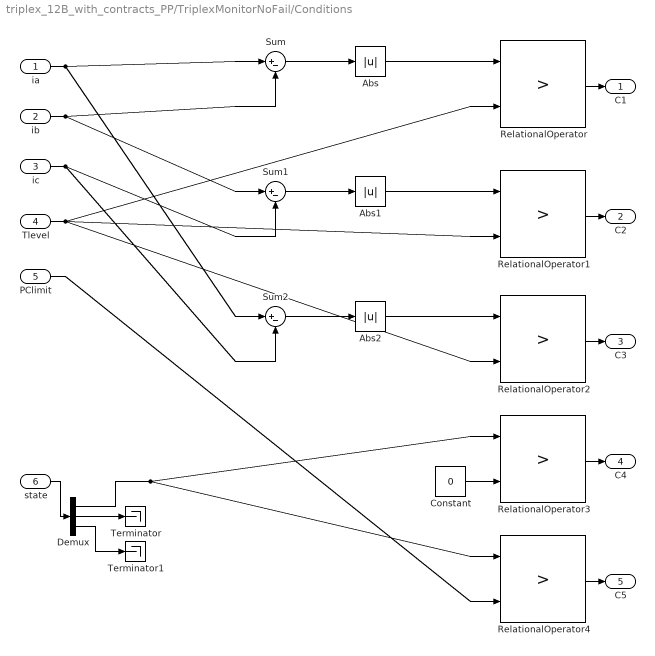
== system triplex_12B_with_contracts_PP/TriplexMonitorNoFail/Conditions ==
  ia : Inport
  ib : Inport  Port=2
  ic : Inport  Port=3
  Tlevel : Inport  Port=4
  PClimit : Inport  Port=5
  state : Inport  Port=6
  Abs : Abs
  Abs1 : Abs
  Abs2 : Abs
  Constant : Constant  Value=0
  Demux : Demux  Outputs=3
  RelationalOperator{,1..4} (5 alike) : RelationalOperator  Operator=>  OutDataTypeStr=boolean  RndMeth=Nearest
  Sum : Sum  Inputs=|+-
  Sum1 : Sum  Inputs=|+-
  Sum2 : Sum  Inputs=|+-
  Terminator : Terminator
  Terminator1 : Terminator
  C1 : Outport  VectorParamsAs1DForOutWhenUnconnected=off
  C2 : Outport  Port=2  VectorParamsAs1DForOutWhenUnconnected=off
  C3 : Outport  Port=3  VectorParamsAs1DForOutWhenUnconnected=off
  C4 : Outport  Port=4  VectorParamsAs1DForOutWhenUnconnected=off
  C5 : Outport  Port=5  VectorParamsAs1DForOutWhenUnconnected=off
  wires:
  Abs/1 -> RelationalOperator/1
  Sum/1 -> Abs/1
  Tlevel/1 -> RelationalOperator/2, RelationalOperator1/2, RelationalOperator2/2
  Constant/1 -> RelationalOperator3/2
  Abs1/1 -> RelationalOperator1/1
  Sum1/1 -> Abs1/1
  Sum2/1 -> Abs2/1
  Abs2/1 -> RelationalOperator2/1
  RelationalOperator4/1 -> C5/1
  ia/1 -> Sum/1, Sum2/1
  RelationalOperator1/1 -> C2/1
  Demux/1 -> RelationalOperator4/1, RelationalOperator3/1
  ic/1 -> Sum1/2, Sum2/2
  RelationalOperator2/1 -> C3/1
  ib/1 -> Sum1/1, Sum/2
  RelationalOperator3/1 -> C4/1
  PClimit/1 -> RelationalOperator4/2
  RelationalOperator/1 -> C1/1
  state/1 -> Demux/1
  Demux/2 -> Terminator/1
  Demux/3 -> Terminator1/1

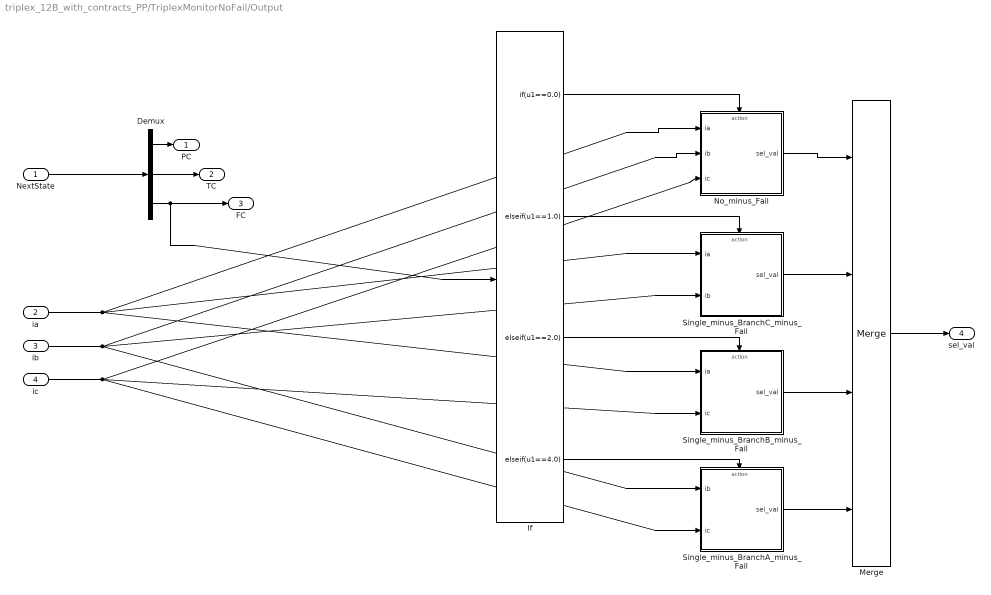
== system triplex_12B_with_contracts_PP/TriplexMonitorNoFail/Output ==
  NextState : Inport
  ia : Inport  Port=2
  ib : Inport  Port=3
  ic : Inport  Port=4
  Demux : Demux  Outputs=3
  If : If  IfExpression=u1==0.0  ElseIfExpressions=u1==1.0, u1==2.0, u1==4.0  ShowElse=off
  Merge : Merge  Inputs=4
  No_minus_Fail : Subsystem  TreatAsAtomicUnit=on
  Single_minus_BranchA_minus_Fail : Subsystem  TreatAsAtomicUnit=on
  Single_minus_BranchB_minus_Fail : Subsystem  TreatAsAtomicUnit=on
  Single_minus_BranchC_minus_Fail : Subsystem  TreatAsAtomicUnit=on
  PC : Outport  VectorParamsAs1DForOutWhenUnconnected=off
  TC : Outport  Port=2  VectorParamsAs1DForOutWhenUnconnected=off
  FC : Outport  Port=3  VectorParamsAs1DForOutWhenUnconnected=off
  sel_val : Outport  Port=4  VectorParamsAs1DForOutWhenUnconnected=off
  wires:
  NextState/1 -> Demux/1
  Demux/1 -> PC/1
  Demux/2 -> TC/1
  Demux/3 -> FC/1, If/1
  If/1 -> No_minus_Fail/Action
  Merge/1 -> sel_val/1
  If/2 -> Single_minus_BranchC_minus_Fail/Action
  ib/1 -> Single_minus_BranchC_minus_Fail/2(ib), No_minus_Fail/2(ib), Single_minus_BranchA_minus_Fail/1(ib)
  If/3 -> Single_minus_BranchB_minus_Fail/Action
  ia/1 -> Single_minus_BranchB_minus_Fail/1(ia), Single_minus_BranchC_minus_Fail/1(ia), No_minus_Fail/1(ia)
  If/4 -> Single_minus_BranchA_minus_Fail/Action
  ic/1 -> Single_minus_BranchA_minus_Fail/2(ic), No_minus_Fail/3(ic), Single_minus_BranchB_minus_Fail/2(ic)
  No_minus_Fail/1(sel_val) -> Merge/1
  Single_minus_BranchC_minus_Fail/1(sel_val) -> Merge/2
  Single_minus_BranchB_minus_Fail/1(sel_val) -> Merge/3
  Single_minus_BranchA_minus_Fail/1(sel_val) -> Merge/4

== system triplex_12B_with_contracts_PP/triplex_12B_TriplexSignalMonitorSpec/TSM_minus_001 ==
  In1 : Inport
  guarantee : Outport  OutDataTypeStr=boolean
  wires:
  In1/1 -> guarantee/1

== system triplex_12B_with_contracts_PP/triplex_12B_TriplexSignalMonitorSpec/TSM_minus_002 ==
  In1 : Inport
  guarantee : Outport  OutDataTypeStr=boolean
  wires:
  In1/1 -> guarantee/1

== system triplex_12B_with_contracts_PP/triplex_12B_TriplexSignalMonitorSpec/TSM_minus_003a ==
  In1 : Inport
  guarantee : Outport  OutDataTypeStr=boolean
  wires:
  In1/1 -> guarantee/1

== system triplex_12B_with_contracts_PP/triplex_12B_TriplexSignalMonitorSpec/TSM_minus_003b ==
  In1 : Inport
  guarantee : Outport  OutDataTypeStr=boolean
  wires:
  In1/1 -> guarantee/1

== system triplex_12B_with_contracts_PP/triplex_12B_TriplexSignalMonitorSpec/TSM_minus_003c ==
  In1 : Inport
  guarantee : Outport  OutDataTypeStr=boolean
  wires:
  In1/1 -> guarantee/1

== system triplex_12B_with_contracts_PP/triplex_12B_TriplexSignalMonitorSpec/TSM_minus_004 ==
  In1 : Inport
  guarantee : Outport  OutDataTypeStr=boolean
  wires:
  In1/1 -> guarantee/1

== system triplex_12B_with_contracts_PP/triplex_12B_TriplexSignalMonitorSpec/abs_call ==
  abs_x : Inport  OutDataTypeStr=double
  branch_6_IF : Switch  Criteria=u2 ~= 0
  xxabs_1_operator : RelationalOperator  OutDataTypeStr=boolean  RndMeth=Simplest
  xxabs_1_rhs_2 : Constant  Value=0.0  OutDataTypeStr=double
  xxabs_2_operator : Gain  Gain=-1  OutDataTypeStr=double
  abs_y : Outport
  wires:
  branch_6_IF/1 -> abs_y/1
  xxabs_1_rhs_2/1 -> xxabs_1_operator/2
  xxabs_2_operator/1 -> branch_6_IF/3
  xxabs_1_operator/1 -> branch_6_IF/2
  abs_x/1 -> xxabs_2_operator/1, xxabs_1_operator/1, branch_6_IF/1

== system triplex_12B_with_contracts_PP/triplex_12B_TriplexSignalMonitorSpec/abs_call1 ==
  abs_x : Inport  OutDataTypeStr=double
  branch_6_IF : Switch  Criteria=u2 ~= 0
  xxabs_1_operator : RelationalOperator  OutDataTypeStr=boolean  RndMeth=Simplest
  xxabs_1_rhs_2 : Constant  Value=0.0  OutDataTypeStr=double
  xxabs_2_operator : Gain  Gain=-1  OutDataTypeStr=double
  abs_y : Outport
  wires:
  branch_6_IF/1 -> abs_y/1
  xxabs_1_rhs_2/1 -> xxabs_1_operator/2
  xxabs_2_operator/1 -> branch_6_IF/3
  xxabs_1_operator/1 -> branch_6_IF/2
  abs_x/1 -> xxabs_2_operator/1, xxabs_1_operator/1, branch_6_IF/1

== system triplex_12B_with_contracts_PP/triplex_12B_TriplexSignalMonitorSpec/abs_call11 ==
  abs_x : Inport  OutDataTypeStr=double
  branch_6_IF : Switch  Criteria=u2 ~= 0
  xxabs_1_operator : RelationalOperator  OutDataTypeStr=boolean  RndMeth=Simplest
  xxabs_1_rhs_2 : Constant  Value=0.0  OutDataTypeStr=double
  xxabs_2_operator : Gain  Gain=-1  OutDataTypeStr=double
  abs_y : Outport
  wires:
  branch_6_IF/1 -> abs_y/1
  xxabs_1_rhs_2/1 -> xxabs_1_operator/2
  xxabs_2_operator/1 -> branch_6_IF/3
  xxabs_1_operator/1 -> branch_6_IF/2
  abs_x/1 -> xxabs_2_operator/1, xxabs_1_operator/1, branch_6_IF/1

== system triplex_12B_with_contracts_PP/triplex_12B_TriplexSignalMonitorSpec/spec284_operator ==
  A : Inport
  B : Inport  Port=2
  Logical_newline_Operator : Logic  Operator=OR  AllPortsSameDT=off  OutDataTypeStr=boolean
  Logical_newline_Operator1 : Logic  Operator=NOT  AllPortsSameDT=off  OutDataTypeStr=boolean
  A_equal__equal__gt_B : Outport  VectorParamsAs1DForOutWhenUnconnected=off
  wires:
  B/1 -> Logical_newline_Operator/2
  A/1 -> Logical_newline_Operator1/1
  Logical_newline_Operator/1 -> A_equal__equal__gt_B/1
  Logical_newline_Operator1/1 -> Logical_newline_Operator/1

== system triplex_12B_with_contracts_PP/triplex_12B_TriplexSignalMonitorSpec/spec292_operator ==
  A : Inport
  B : Inport  Port=2
  Logical_newline_Operator : Logic  Operator=OR  AllPortsSameDT=off  OutDataTypeStr=boolean
  Logical_newline_Operator1 : Logic  Operator=NOT  AllPortsSameDT=off  OutDataTypeStr=boolean
  A_equal__equal__gt_B : Outport  VectorParamsAs1DForOutWhenUnconnected=off
  wires:
  B/1 -> Logical_newline_Operator/2
  A/1 -> Logical_newline_Operator1/1
  Logical_newline_Operator/1 -> A_equal__equal__gt_B/1
  Logical_newline_Operator1/1 -> Logical_newline_Operator/1

== system triplex_12B_with_contracts_PP/triplex_12B_TriplexSignalMonitorSpec/spec309_operator ==
  A : Inport
  B : Inport  Port=2
  Logical_newline_Operator : Logic  Operator=OR  AllPortsSameDT=off  OutDataTypeStr=boolean
  Logical_newline_Operator1 : Logic  Operator=NOT  AllPortsSameDT=off  OutDataTypeStr=boolean
  A_equal__equal__gt_B : Outport  VectorParamsAs1DForOutWhenUnconnected=off
  wires:
  B/1 -> Logical_newline_Operator/2
  A/1 -> Logical_newline_Operator1/1
  Logical_newline_Operator/1 -> A_equal__equal__gt_B/1
  Logical_newline_Operator1/1 -> Logical_newline_Operator/1

== system triplex_12B_with_contracts_PP/triplex_12B_TriplexSignalMonitorSpec/spec326_operator ==
  A : Inport
  B : Inport  Port=2
  Logical_newline_Operator : Logic  Operator=OR  AllPortsSameDT=off  OutDataTypeStr=boolean
  Logical_newline_Operator1 : Logic  Operator=NOT  AllPortsSameDT=off  OutDataTypeStr=boolean
  A_equal__equal__gt_B : Outport  VectorParamsAs1DForOutWhenUnconnected=off
  wires:
  B/1 -> Logical_newline_Operator/2
  A/1 -> Logical_newline_Operator1/1
  Logical_newline_Operator/1 -> A_equal__equal__gt_B/1
  Logical_newline_Operator1/1 -> Logical_newline_Operator/1

== system triplex_12B_with_contracts_PP/triplex_12B_TriplexSignalMonitorSpec/spec334_operator ==
  A : Inport
  B : Inport  Port=2
  Logical_newline_Operator : Logic  Operator=OR  AllPortsSameDT=off  OutDataTypeStr=boolean
  Logical_newline_Operator1 : Logic  Operator=NOT  AllPortsSameDT=off  OutDataTypeStr=boolean
  A_equal__equal__gt_B : Outport  VectorParamsAs1DForOutWhenUnconnected=off
  wires:
  B/1 -> Logical_newline_Operator/2
  A/1 -> Logical_newline_Operator1/1
  Logical_newline_Operator/1 -> A_equal__equal__gt_B/1
  Logical_newline_Operator1/1 -> Logical_newline_Operator/1

== system triplex_12B_with_contracts_PP/triplex_12B_TriplexSignalMonitorSpec/spec351_operator ==
  A : Inport
  B : Inport  Port=2
  Logical_newline_Operator : Logic  Operator=OR  AllPortsSameDT=off  OutDataTypeStr=boolean
  Logical_newline_Operator1 : Logic  Operator=NOT  AllPortsSameDT=off  OutDataTypeStr=boolean
  A_equal__equal__gt_B : Outport  VectorParamsAs1DForOutWhenUnconnected=off
  wires:
  B/1 -> Logical_newline_Operator/2
  A/1 -> Logical_newline_Operator1/1
  Logical_newline_Operator/1 -> A_equal__equal__gt_B/1
  Logical_newline_Operator1/1 -> Logical_newline_Operator/1

== system triplex_12B_with_contracts_PP/TriplexMonitorNoFail/Actions/Act1 ==
  note: // Action 1: No pending failures
  state : Inport
  ActionPort : ActionPort  ActionPortLabel=if(u1)
  Constant1 : Constant  Value=0  OutDataTypeStr=int32
  Demux : Demux  Outputs=3
  Mux : Mux  Inputs=3
  SignalConversion : SignalConversion  OverrideOpt=off
  Terminator : Terminator
  NextState : Outport  VectorParamsAs1DForOutWhenUnconnected=off
  wires:
  SignalConversion/1 -> NextState/1
  Mux/1 -> SignalConversion/1
  state/1 -> Demux/1
  Demux/2 -> Mux/2
  Demux/3 -> Mux/3
  Constant1/1 -> Mux/1
  Demux/1 -> Terminator/1

== system triplex_12B_with_contracts_PP/TriplexMonitorNoFail/Actions/Act2 ==
  note: // Action 2: Failure pending but no miscompares
  state : Inport
  ActionPort : ActionPort  ActionPortLabel=elseif(u2)
  Constant1 : Constant  OutDataTypeStr=int32
  Demux : Demux  Outputs=3
  Mux : Mux  Inputs=3
  SignalConversion : SignalConversion  OverrideOpt=off
  Sum : Sum  Inputs=-+|
  NextState : Outport  VectorParamsAs1DForOutWhenUnconnected=off
  wires:
  Constant1/1 -> Sum/1
  SignalConversion/1 -> NextState/1
  Mux/1 -> SignalConversion/1
  state/1 -> Demux/1
  Demux/2 -> Mux/2
  Demux/3 -> Mux/3
  Sum/1 -> Mux/1
  Demux/1 -> Sum/2

== system triplex_12B_with_contracts_PP/TriplexMonitorNoFail/Actions/Act3 ==
  note: // Action 3: Do nothing there is only 1 miscompare
  state : Inport
  ActionPort : ActionPort  ActionPortLabel=elseif( u3)
  NextState : Outport  VectorParamsAs1DForOutWhenUnconnected=off
  wires:
  state/1 -> NextState/1

== system triplex_12B_with_contracts_PP/TriplexMonitorNoFail/Actions/Act4 ==
  note: // Action 4: Failure pending
  state : Inport
  ActionPort : ActionPort  ActionPortLabel=elseif( u4)
  Constant1 : Constant  OutDataTypeStr=int32
  Demux : Demux  Outputs=3
  Mux : Mux  Inputs=3
  SignalConversion : SignalConversion  OverrideOpt=off
  Sum : Sum  Inputs=++|
  Sum1 : Sum  Inputs=|++
  NextState : Outport  VectorParamsAs1DForOutWhenUnconnected=off
  wires:
  SignalConversion/1 -> NextState/1
  Mux/1 -> SignalConversion/1
  state/1 -> Demux/1
  Demux/2 -> Sum/2
  Constant1/1 -> Sum1/2, Sum/1
  Demux/1 -> Sum1/1
  Sum1/1 -> Mux/1
  Sum/1 -> Mux/2
  Demux/3 -> Mux/3

== system triplex_12B_with_contracts_PP/TriplexMonitorNoFail/Actions/Act5 ==
  note: // Action 5: Failure latched (branch B)
  state : Inport
  ActionPort : ActionPort  ActionPortLabel=elseif( u5)
  Constant : Constant  Value=0  OutDataTypeStr=int32
  Constant1 : Constant  Value=2  OutDataTypeStr=int32
  Mux : Mux  Inputs=3
  Selector : Selector  InputPortWidth=3  IndexOptions=Index vector (dialog)  Indices=[2]  OutputSizes=1
  SignalConversion : SignalConversion  OverrideOpt=off
  NextState : Outport  VectorParamsAs1DForOutWhenUnconnected=off
  wires:
  Mux/1 -> SignalConversion/1
  Constant/1 -> Mux/1
  Constant1/1 -> Mux/3
  Selector/1 -> Mux/2
  state/1 -> Selector/1
  SignalConversion/1 -> NextState/1

== system triplex_12B_with_contracts_PP/TriplexMonitorNoFail/Actions/Act6 ==
  note: // Action 6: Failure latched (branch A)
  state : Inport
  ActionPort : ActionPort  ActionPortLabel=elseif( u6)
  Constant : Constant  Value=0  OutDataTypeStr=int32
  Constant1 : Constant  Value=4  OutDataTypeStr=int32
  Mux : Mux  Inputs=3
  Selector : Selector  InputPortWidth=3  IndexOptions=Index vector (dialog)  Indices=[2]  OutputSizes=1
  SignalConversion : SignalConversion  OverrideOpt=off
  NextState : Outport  VectorParamsAs1DForOutWhenUnconnected=off
  wires:
  Mux/1 -> SignalConversion/1
  Constant/1 -> Mux/1
  Constant1/1 -> Mux/3
  Selector/1 -> Mux/2
  state/1 -> Selector/1
  SignalConversion/1 -> NextState/1

== system triplex_12B_with_contracts_PP/TriplexMonitorNoFail/Actions/Act7 ==
  note: /// Action 7: Failure latched (branch C)
  state : Inport
  ActionPort : ActionPort  ActionPortLabel=elseif( u7)
  Constant : Constant  Value=0  OutDataTypeStr=int32
  Constant1 : Constant  OutDataTypeStr=int32
  Mux : Mux  Inputs=3
  Selector : Selector  InputPortWidth=3  IndexOptions=Index vector (dialog)  Indices=[2]  OutputSizes=1
  SignalConversion : SignalConversion  OverrideOpt=off
  NextState : Outport  VectorParamsAs1DForOutWhenUnconnected=off
  wires:
  Mux/1 -> SignalConversion/1
  Constant/1 -> Mux/1
  Constant1/1 -> Mux/3
  Selector/1 -> Mux/2
  state/1 -> Selector/1
  SignalConversion/1 -> NextState/1

== system triplex_12B_with_contracts_PP/TriplexMonitorNoFail/Actions/Act8 ==
  note: // Action 8: All branches miscompare
  state : Inport
  ActionPort : ActionPort  ActionPortLabel=elseif( u8)
  Constant1 : Constant  OutDataTypeStr=int32
  Demux : Demux  Outputs=3
  Mux : Mux  Inputs=3
  SignalConversion : SignalConversion  OverrideOpt=off
  Sum1 : Sum  Inputs=++|
  NextState : Outport  VectorParamsAs1DForOutWhenUnconnected=off
  wires:
  Mux/1 -> SignalConversion/1
  Demux/1 -> Mux/1
  Demux/3 -> Mux/3
  Sum1/1 -> Mux/2
  Constant1/1 -> Sum1/1
  Demux/2 -> Sum1/2
  SignalConversion/1 -> NextState/1
  state/1 -> Demux/1

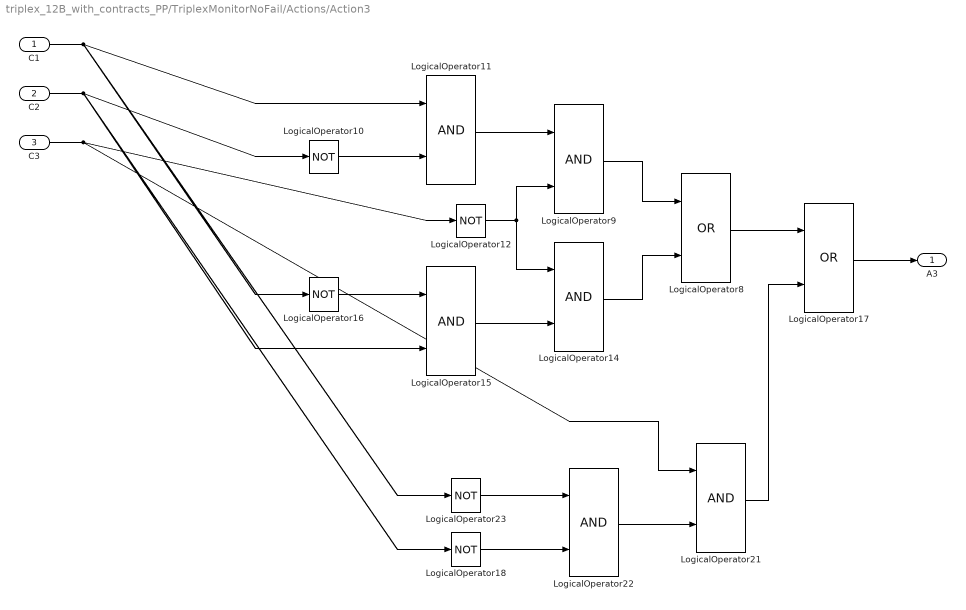
== system triplex_12B_with_contracts_PP/TriplexMonitorNoFail/Actions/Action3 ==
  C1 : Inport
  C2 : Inport  Port=2
  C3 : Inport  Port=3
  LogicalOperator{10,12,16,18,23} (5 alike) : Logic  Operator=NOT  Inputs=1  AllPortsSameDT=off  OutDataTypeStr=boolean
  LogicalOperator{9,11,14..15,21..22} (6 alike) : Logic  AllPortsSameDT=off  OutDataTypeStr=boolean
  LogicalOperator17 : Logic  Operator=OR  AllPortsSameDT=off  OutDataTypeStr=boolean
  LogicalOperator8 : Logic  Operator=OR  AllPortsSameDT=off  OutDataTypeStr=boolean
  A3 : Outport  VectorParamsAs1DForOutWhenUnconnected=off
  wires:
  LogicalOperator10/1 -> LogicalOperator11/2
  LogicalOperator12/1 -> LogicalOperator9/2, LogicalOperator14/1
  LogicalOperator11/1 -> LogicalOperator9/1
  LogicalOperator16/1 -> LogicalOperator15/1
  LogicalOperator9/1 -> LogicalOperator8/1
  C2/1 -> LogicalOperator15/2, LogicalOperator18/1, LogicalOperator10/1
  LogicalOperator15/1 -> LogicalOperator14/2
  LogicalOperator14/1 -> LogicalOperator8/2
  LogicalOperator8/1 -> LogicalOperator17/1
  LogicalOperator21/1 -> LogicalOperator17/2
  C1/1 -> LogicalOperator23/1, LogicalOperator11/1, LogicalOperator16/1
  C3/1 -> LogicalOperator21/1, LogicalOperator12/1
  LogicalOperator23/1 -> LogicalOperator22/1
  LogicalOperator22/1 -> LogicalOperator21/2
  LogicalOperator18/1 -> LogicalOperator22/2
  LogicalOperator17/1 -> A3/1

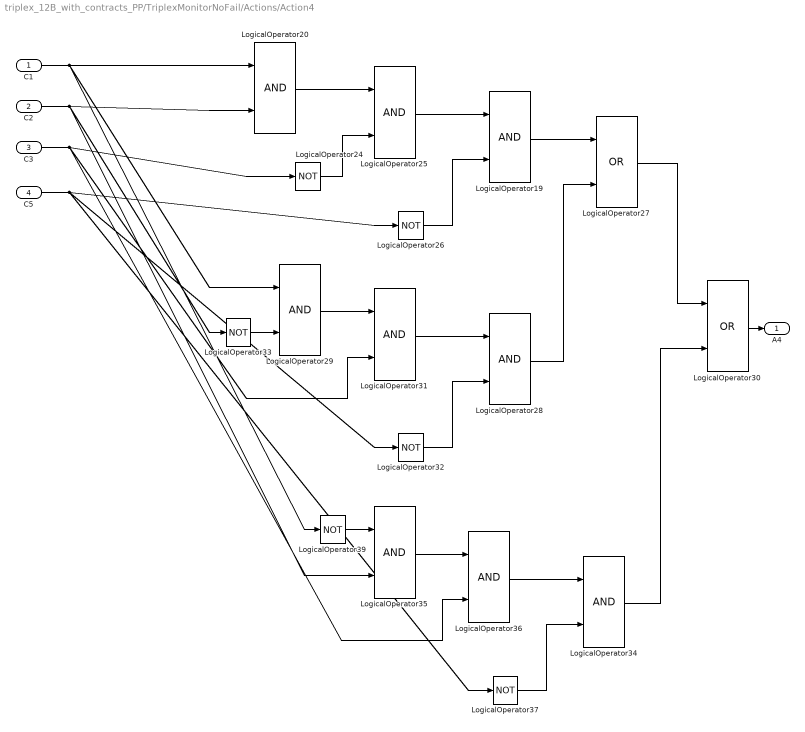
== system triplex_12B_with_contracts_PP/TriplexMonitorNoFail/Actions/Action4 ==
  C1 : Inport
  C2 : Inport  Port=2
  C3 : Inport  Port=3
  C5 : Inport  Port=4
  LogicalOperator{19..20,25,28..29,31,34..36} (9 alike) : Logic  AllPortsSameDT=off  OutDataTypeStr=boolean
  LogicalOperator{24,26,32..33,37,39} (6 alike) : Logic  Operator=NOT  Inputs=1  AllPortsSameDT=off  OutDataTypeStr=boolean
  LogicalOperator27 : Logic  Operator=OR  AllPortsSameDT=off  OutDataTypeStr=boolean
  LogicalOperator30 : Logic  Operator=OR  AllPortsSameDT=off  OutDataTypeStr=boolean
  A4 : Outport  VectorParamsAs1DForOutWhenUnconnected=off
  wires:
  LogicalOperator31/1 -> LogicalOperator28/1
  LogicalOperator32/1 -> LogicalOperator28/2
  LogicalOperator28/1 -> LogicalOperator27/2
  LogicalOperator29/1 -> LogicalOperator31/1
  C3/1 -> LogicalOperator24/1, LogicalOperator31/2, LogicalOperator36/2
  C2/1 -> LogicalOperator20/2, LogicalOperator33/1, LogicalOperator35/2
  C1/1 -> LogicalOperator20/1, LogicalOperator29/1, LogicalOperator39/1
  LogicalOperator20/1 -> LogicalOperator25/1
  LogicalOperator30/1 -> A4/1
  LogicalOperator26/1 -> LogicalOperator19/2
  LogicalOperator33/1 -> LogicalOperator29/2
  LogicalOperator25/1 -> LogicalOperator19/1
  C5/1 -> LogicalOperator26/1, LogicalOperator32/1, LogicalOperator37/1
  LogicalOperator19/1 -> LogicalOperator27/1
  LogicalOperator24/1 -> LogicalOperator25/2
  LogicalOperator36/1 -> LogicalOperator34/1
  LogicalOperator27/1 -> LogicalOperator30/1
  LogicalOperator37/1 -> LogicalOperator34/2
  LogicalOperator39/1 -> LogicalOperator35/1
  LogicalOperator35/1 -> LogicalOperator36/1
  LogicalOperator34/1 -> LogicalOperator30/2

== system triplex_12B_with_contracts_PP/TriplexMonitorNoFail/Actions/Action8 ==
  C1 : Inport
  C2 : Inport  Port=2
  C3 : Inport  Port=3
  LogicalOperator3 : Logic  AllPortsSameDT=off  OutDataTypeStr=boolean
  LogicalOperator4 : Logic  AllPortsSameDT=off  OutDataTypeStr=boolean
  A8 : Outport  VectorParamsAs1DForOutWhenUnconnected=off
  wires:
  LogicalOperator3/1 -> LogicalOperator4/1
  C3/1 -> LogicalOperator4/2
  C1/1 -> LogicalOperator3/1
  C2/1 -> LogicalOperator3/2
  LogicalOperator4/1 -> A8/1

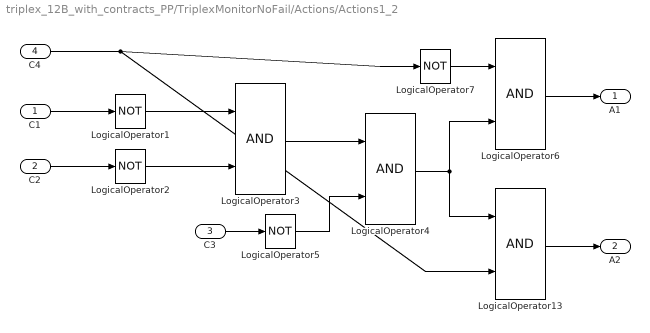
== system triplex_12B_with_contracts_PP/TriplexMonitorNoFail/Actions/Actions1_2 ==
  C1 : Inport
  C2 : Inport  Port=2
  C3 : Inport  Port=3
  C4 : Inport  Port=4
  LogicalOperator{1..2,5,7} (4 alike) : Logic  Operator=NOT  Inputs=1  AllPortsSameDT=off  OutDataTypeStr=boolean
  LogicalOperator{3..4,6,13} (4 alike) : Logic  AllPortsSameDT=off  OutDataTypeStr=boolean
  A1 : Outport  VectorParamsAs1DForOutWhenUnconnected=off
  A2 : Outport  Port=2  VectorParamsAs1DForOutWhenUnconnected=off
  wires:
  C2/1 -> LogicalOperator2/1
  LogicalOperator4/1 -> LogicalOperator6/2, LogicalOperator13/1
  LogicalOperator2/1 -> LogicalOperator3/2
  C1/1 -> LogicalOperator1/1
  LogicalOperator1/1 -> LogicalOperator3/1
  LogicalOperator6/1 -> A1/1
  LogicalOperator7/1 -> LogicalOperator6/1
  LogicalOperator3/1 -> LogicalOperator4/1
  C4/1 -> LogicalOperator7/1, LogicalOperator13/2
  LogicalOperator13/1 -> A2/1
  LogicalOperator5/1 -> LogicalOperator4/2
  C3/1 -> LogicalOperator5/1
